simulink model "Demo_DSRC_DNPW_cs"  (Simulink 7.6)
settings: Solver=ode5  SolverMode=SingleTasking  StartTime=0.0  StopTime=5  FixedStep=1/20  RelTol=1e-3
model workspace (MAT data in the model file):
  mbox_table : struct (value not decoded)
  model_closed = 0
  sim_status = 0
PreLoadFcn:
  | check_NUTS_defined;
  | 
  | assignin('base',['model_closed_' bdroot],false);
InitFcn:
  | PreScanExperimentInitFcn(bdroot)
StopFcn:
  | PreScanExperimentStopFcn(bdroot)
undefined symbols (not defined in the file): DiscIntNeverNeededParam, spare_1, spare_10, spare_11, spare_12, spare_13, spare_14, spare_15, spare_16, spare_17, spare_18, spare_19, spare_2, spare_3, spare_4, spare_5, spare_6, spare_7, spare_8, spare_9
libraries: PreScanSimulinkLibrary x29, PreScanUsefulBlocks x11, simulink x9, simulink_extras x2
(part 1 of 6)
CloseFcn:
  | evalin('base',['clear model_closed_' bdroot]);
settings Model: Creator=PRESCAN  LastModifiedBy=buildbot
settings OptimizationCC: InitFltsAndDblsToZero=on
settings DebuggingCC: SaveWithParameterizedLinksMsg=none  SignalResolutionControl=TryResolveAllWithWarning  SolverPrmCheckMsg=none  MultiTaskDSMMsg=warning  MultiTaskCondExecSysMsg=none
settings SFSimCC: SimParseCustomCode=off
settings RTWCC: IncludeERTFirstTime=on
settings GRTTargetCC: TargetFcnLib=ansi_tfl_tmw.mat

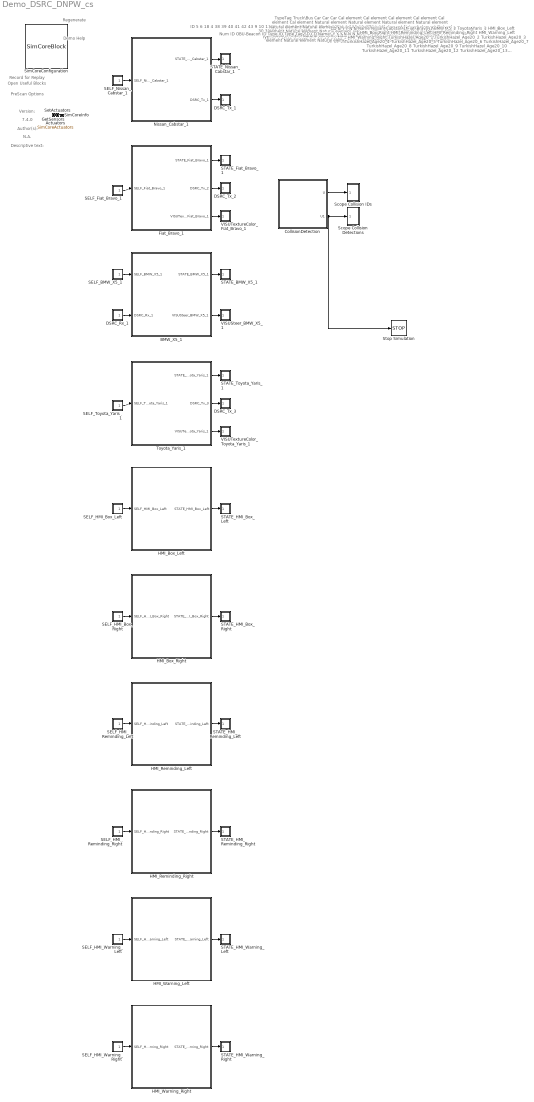
== system Demo_DSRC_DNPW_cs ==
  note: Demo Help
  note: Regenerate
  note: Record for Replay
  note: Open Useful Blocks
  note: PreScan Options
  note: Version:
  note: 7.4.0
  note: Author(s):
  note: N.A.
  note: Descriptive text:
  note: ID
      |
      | 5
      | 6
      | 18
      | 4
      | 38
      | 39
      | 40
      | 41
      | 42
      | 43
      | 9
      | 10
      | 11
      | 12
      | 13
      | 14
      | 15
      | 16
      | 17
      | 19
      | 20
      | 21
      | 22
      | 23
      | 24
      | 25
      | 26
      | 27
      | 28
      | 29
      | 30
      | 31
      | 32
      | 33
      | 34
      | 35
      | 36
      | 37
  note: OBU-Beacon ID
  note: TypeID
      |
      | 3
      | 1
      | 1
      | 1
      | 5
      | 5
      | 5
      | 5
      | 5
      | 5
      | 13
      | 13
      | 13
      | 13
      | 13
      | 13
      | 13
      | 13
      | 13
      | 13
      | 13
      | 13
      | 13
      | 13
      | 13
      | 13
      | 13
      | 13
      | 13
      | 13
      | 13
      | 13
      | 13
      | 13
      | 13
      | 13
      | 13
      | 13
  note: TypeTag
      |
      | Truck\Bus
      | Car
      | Car
      | Car
      | Cal element
      | Cal element
      | Cal element
      | Cal element
      | Cal element
      | Cal element
      | Natural element
      | Natural element
      | Natural element
      | Natural element
      | Natural element
      | Natural element
      | Natural element
      | Natural element
      | Natural element
      | Natural element
      | Natural element
      | Natural element
      | Natural element
      | Natural element
      | Natural element
      | Natural element
      | Natural element
      | Natural element
      | Natural element
      | Natural element
      | Natural element
      | Natural element
      | Natural element
      | Natural element
      | Natural element
      | Natural element
      | Natural element
      | Natural element
  note: SD
      |
      | Y
      | Y
      | Y
      | Y
      | N
      | N
      | N
      | N
      | N
      | N
      | Y
      | Y
      | Y
      | Y
      | Y
      | Y
      | Y
      | Y
      | Y
      | Y
      | Y
      | Y
      | Y
      | Y
      | Y
      | Y
      | Y
      | Y
      | Y
      | Y
      | Y
      | Y
      | Y
      | Y
      | Y
      | Y
      | Y
      | Y
  note: CD
      |
      | N
      | Y
      | Y
      | N
      | N
      | N
      | N
      | N
      | N
      | N
      | N
      | N
      | N
      | N
      | N
      | N
      | N
      | N
      | N
      | N
      | N
      | N
      | N
      | N
      | N
      | N
      | N
      | N
      | N
      | N
      | N
      | N
      | N
      | N
      | N
      | N
      | N
      | N
  note: Name
      |
      | Nissan_Cabstar_1
      | Fiat_Bravo_1
      | BMW_X5_1
      | Toyota_Yaris_1
      | HMI_Box_Left
      | HMI_Box_Right
      | HMI_Reminding_Left
      | HMI_Reminding_Right
      | HMI_Warning_Left
      | HMI_Warning_Right
      | TurkishHazel_Age20_1
      | TurkishHazel_Age20_2
      | TurkishHazel_Age20_3
      | TurkishHazel_Age20_4
      | TurkishHazel_Age20_5
      | TurkishHazel_Age20_6
      | TurkishHazel_Age20_7
      | TurkishHazel_Age20_8
      | TurkishHazel_Age20_9
      | TurkishHazel_Age20_10
      | TurkishHazel_Age20_11
      | TurkishHazel_Age20_12
      | TurkishHazel_Age20_13
      | TurkishHazel_Age20_14
      | TurkishHazel_Age20_15
      | TurkishHazel_Age20_16
      | TurkishHazel_Age20_17
      | TurkishHazel_Age20_18
      | TurkishHazel_Age20_19
      | TurkishHazel_Age20_20
      | TurkishHazel_Age20_21
      | TurkishHazel_Age20_22
      | TurkishHazel_Age20_23
      | TurkishHazel_Age20_24
      | TurkishHazel_Age20_25
      | TurkishHazel_Age20_26
      | TurkishHazel_Age20_27
      | TurkishHazel_Age20_28
  note: Num ID OBU-Beacon ID Type ID Type Tag SD CD Name
  Actuators : DataStoreMemory  Tag=Actuators  DataStoreName=SimCoreActuators  InitialValue=zeros(236,1)
      settings: DeleteFcn=PreScanBlockDeleteFcn;
  BMW_X5_1 : Subsystem  Tag=WorldObjectSubSystem  InitFcn=UniqueId = '51';
      mask Display: image(imread('BMW_X5.jpg'));color('white');text(0,0,' ID=18\n')
  CollisionDetection : Subsystem  Tag=CollisionDetection  Priority=3  mask(PreScan Source Block: CollisionDetection){PortName=CollisionDetection, PortIndex=0, PortWidth=10, TimeStep=1/20}
      mask prompts: PortName "Auto-Assigned: Port Name [-]"; PortIndex "Auto-Assigned: Port Index [-]"; PortWidth "Auto-Assigned: Port Dimensions"; TimeStep "Auto-Assigned: Upload Period [s]"
      mask help:
      | The SELF port shows (state) information of the actor itself. The outputs are position in the experiment's axis system and the GPS coordinates, and the object's absolute velocity and compass heading.
      |
      | For more information, please click Help.
      settings: DeleteFcn=PreScanBlockDeleteFcn;
      mask Help: eval('openHelp(811)')
      mask Display: image(imread('crash.jpg'))
  DSRC_Rx_1 : Subsystem  Tag=DSRC_R  Priority=3  mask(PreScan Source Block: DSRC Receiver){NrEntitiesOut=3, PortName=DSRC_Rx_1, PortIndex=34, PortWidth=141, TimeStep=1/20}
      mask prompts: NrEntitiesOut "User Specified: # of Visible Actors"; PortName "Auto Assigned: Port Name [-]"; PortIndex "Auto Assigned: Index [-]"; PortWidth "Auto Assigned: Port Dimensions [-]"; TimeStep "Auto Assigned: Upload Period [s]"
      mask help:
      | Using the DSRC Receiver (R) and Transmitter (T) information between actors can be exchanged.
      |
      | The DSRC Reciever receives actor information.
      |
      | For more information, please click Help.
      settings: DeleteFcn=PreScanBlockDeleteFcn;
      mask Help: eval('openHelp(473)')
      mask Display: image(imread('DSRCReceiver.png'))
  DSRC_Tx_1 : Subsystem  Tag=DSRC_T  Priority=0  mask(PreScan Sink Block: DSRC_T){PortName=DSRC_Tx_1, PortIndex=15, PortWidth=24, TimeStep=1/20}
      mask prompts: PortName "Auto Assigned: Port Name [-]"; PortIndex "Auto Assigned: Index [-]"; PortWidth "Auto Assigned: Port Dimensions [-]"; TimeStep "Auto Assigned: Upload Period [s]"
      mask help:
      | Using the DSRC Receiver and Transmitter information between actors can be exchanged.
      |
      | The DSRC Transmitter receives actors information.
      |
      | For more information, please click Help.
      settings: DeleteFcn=PreScanBlockDeleteFcn;
      mask Help: eval('openHelp(473)')
      mask Display: image(imread('DSRCTransmitter.png'))
  DSRC_Tx_2 : Subsystem  Tag=DSRC_T  Priority=0  mask(PreScan Sink Block: DSRC_T){PortName=DSRC_Tx_2, PortIndex=54, PortWidth=24, TimeStep=1/20}
      mask prompts: PortName "Auto Assigned: Port Name [-]"; PortIndex "Auto Assigned: Index [-]"; PortWidth "Auto Assigned: Port Dimensions [-]"; TimeStep "Auto Assigned: Upload Period [s]"
      mask help:
      | Using the DSRC Receiver and Transmitter information between actors can be exchanged.
      |
      | The DSRC Transmitter receives actors information.
      |
      | For more information, please click Help.
      settings: DeleteFcn=PreScanBlockDeleteFcn;
      mask Help: eval('openHelp(473)')
      mask Display: image(imread('DSRCTransmitter.png'))
  DSRC_Tx_3 : Subsystem  Tag=DSRC_T  Priority=0  mask(PreScan Sink Block: DSRC_T){PortName=DSRC_Tx_3, PortIndex=119, PortWidth=24, TimeStep=1/20}
      mask prompts: PortName "Auto Assigned: Port Name [-]"; PortIndex "Auto Assigned: Index [-]"; PortWidth "Auto Assigned: Port Dimensions [-]"; TimeStep "Auto Assigned: Upload Period [s]"
      mask help:
      | Using the DSRC Receiver and Transmitter information between actors can be exchanged.
      |
      | The DSRC Transmitter receives actors information.
      |
      | For more information, please click Help.
      settings: DeleteFcn=PreScanBlockDeleteFcn;
      mask Help: eval('openHelp(473)')
      mask Display: image(imread('DSRCTransmitter.png'))
  Fiat_Bravo_1 : Subsystem  Tag=WorldObjectSubSystem  InitFcn=UniqueId = '21';
      mask Display: image(imread('Fiat_Bravo.jpg'));color('white');text(0,0,' ID=6\n')
  GetSensors : Subsystem  Tag=GetSensors  Priority=2  mask(PreScan Simulation Core Block){NrOfSensors=231, TimeStep=1/20}
      mask prompts: NrOfSensors "Number of sensor values"; TimeStep "Timestep [s]"
      mask help:
      | Please do not remove this block from the PreScan compilation sheet,
      | as it contains essential configuration parameters for a PreScan simulation.
      settings: DeleteFcn=PreScanBlockDeleteFcn;
  HMI_Box_Left : Subsystem  Tag=WorldObjectSubSystem  InitFcn=UniqueId = '84';
      mask Display: image(imread('Box.jpg'));color('white');text(0,0,' ID=38\n')
  HMI_Box_Right : Subsystem  Tag=WorldObjectSubSystem  InitFcn=UniqueId = '85';
      mask Display: image(imread('Box.jpg'));color('white');text(0,0,' ID=39\n')
  HMI_Reminding_Left : Subsystem  Tag=WorldObjectSubSystem  InitFcn=UniqueId = '86';
      mask Display: image(imread('Sphere.jpg'));color('white');text(0,0,' ID=40\n')
  HMI_Reminding_Right : Subsystem  Tag=WorldObjectSubSystem  InitFcn=UniqueId = '87';
      mask Display: image(imread('Sphere.jpg'));color('white');text(0,0,' ID=41\n')
  HMI_Warning_Left : Subsystem  Tag=WorldObjectSubSystem  InitFcn=UniqueId = '88';
      mask Display: image(imread('Sphere.jpg'));color('white');text(0,0,' ID=42\n')
  HMI_Warning_Right : Subsystem  Tag=WorldObjectSubSystem  InitFcn=UniqueId = '89';
      mask Display: image(imread('Sphere.jpg'));color('white');text(0,0,' ID=43\n')
  Nissan_Cabstar_1 : Subsystem  Tag=WorldObjectSubSystem  InitFcn=UniqueId = '19';
      mask Display: image(imread('Nissan_Cabstar.jpg'));color('white');text(0,0,' ID=5\n')
  SELF_BMW_X5_1 : Subsystem  Tag=SELF  Priority=3  mask(PreScan Source Block: SELF){PortName=SELF_BMW_X5_1, PortIndex=26, PortWidth=8, TimeStep=1/20}
      mask prompts: PortName "Auto-Assigned: Port Name [-]"; PortIndex "Auto-Assigned: Port Index [-]"; PortWidth "Auto-Assigned: Port Dimensions"; TimeStep "Auto-Assigned: Upload Period [s]"
      mask help:
      | The SELF port shows (state) information of the actor itself. The outputs are position in the experiment's axis system and the GPS coordinates, and the object's absolute velocity and compass heading.
      |
      | For more information, please click Help.
      settings: DeleteFcn=PreScanBlockDeleteFcn;
      mask Help: eval('openHelp(462)')
      mask Display: image(imread('GPS.png'))
  SELF_Fiat_Bravo_1 : Subsystem  Tag=SELF  Priority=3  mask(PreScan Source Block: SELF){PortName=SELF_Fiat_Bravo_1, PortIndex=18, PortWidth=8, TimeStep=1/20}
      mask prompts: PortName "Auto-Assigned: Port Name [-]"; PortIndex "Auto-Assigned: Port Index [-]"; PortWidth "Auto-Assigned: Port Dimensions"; TimeStep "Auto-Assigned: Upload Period [s]"
      mask help:
      | The SELF port shows (state) information of the actor itself. The outputs are position in the experiment's axis system and the GPS coordinates, and the object's absolute velocity and compass heading.
      |
      | For more information, please click Help.
      settings: DeleteFcn=PreScanBlockDeleteFcn;
      mask Help: eval('openHelp(462)')
      mask Display: image(imread('GPS.png'))
  SELF_HMI_Box_Left : Subsystem  Tag=SELF  Priority=3  mask(PreScan Source Block: SELF){PortName=SELF_HMI_Box_Left, PortIndex=183, PortWidth=8, TimeStep=1/20}
      mask prompts: PortName "Auto-Assigned: Port Name [-]"; PortIndex "Auto-Assigned: Port Index [-]"; PortWidth "Auto-Assigned: Port Dimensions"; TimeStep "Auto-Assigned: Upload Period [s]"
      mask help:
      | The SELF port shows (state) information of the actor itself. The outputs are position in the experiment's axis system and the GPS coordinates, and the object's absolute velocity and compass heading.
      |
      | For more information, please click Help.
      settings: DeleteFcn=PreScanBlockDeleteFcn;
      mask Help: eval('openHelp(462)')
      mask Display: image(imread('GPS.png'))
  SELF_HMI_Box_Right : Subsystem  Tag=SELF  Priority=3  mask(PreScan Source Block: SELF){PortName=SELF_HMI_Box_Right, PortIndex=191, PortWidth=8, TimeStep=1/20}
      mask prompts: PortName "Auto-Assigned: Port Name [-]"; PortIndex "Auto-Assigned: Port Index [-]"; PortWidth "Auto-Assigned: Port Dimensions"; TimeStep "Auto-Assigned: Upload Period [s]"
      mask help:
      | The SELF port shows (state) information of the actor itself. The outputs are position in the experiment's axis system and the GPS coordinates, and the object's absolute velocity and compass heading.
      |
      | For more information, please click Help.
      settings: DeleteFcn=PreScanBlockDeleteFcn;
      mask Help: eval('openHelp(462)')
      mask Display: image(imread('GPS.png'))
  SELF_HMI_Reminding_Left : Subsystem  Tag=SELF  Priority=3  mask(PreScan Source Block: SELF){PortName=SELF_HMI_Reminding_Left, PortIndex=199, PortWidth=8, TimeStep=1/20}
      mask prompts: PortName "Auto-Assigned: Port Name [-]"; PortIndex "Auto-Assigned: Port Index [-]"; PortWidth "Auto-Assigned: Port Dimensions"; TimeStep "Auto-Assigned: Upload Period [s]"
      mask help:
      | The SELF port shows (state) information of the actor itself. The outputs are position in the experiment's axis system and the GPS coordinates, and the object's absolute velocity and compass heading.
      |
      | For more information, please click Help.
      settings: DeleteFcn=PreScanBlockDeleteFcn;
      mask Help: eval('openHelp(462)')
      mask Display: image(imread('GPS.png'))
  SELF_HMI_Reminding_Right : Subsystem  Tag=SELF  Priority=3  mask(PreScan Source Block: SELF){PortName=SELF_HMI_Reminding_Right, PortIndex=207, PortWidth=8, TimeStep=1/20}
      mask prompts: PortName "Auto-Assigned: Port Name [-]"; PortIndex "Auto-Assigned: Port Index [-]"; PortWidth "Auto-Assigned: Port Dimensions"; TimeStep "Auto-Assigned: Upload Period [s]"
      mask help:
      | The SELF port shows (state) information of the actor itself. The outputs are position in the experiment's axis system and the GPS coordinates, and the object's absolute velocity and compass heading.
      |
      | For more information, please click Help.
      settings: DeleteFcn=PreScanBlockDeleteFcn;
      mask Help: eval('openHelp(462)')
      mask Display: image(imread('GPS.png'))
  SELF_HMI_Warning_Left : Subsystem  Tag=SELF  Priority=3  mask(PreScan Source Block: SELF){PortName=SELF_HMI_Warning_Left, PortIndex=215, PortWidth=8, TimeStep=1/20}
      mask prompts: PortName "Auto-Assigned: Port Name [-]"; PortIndex "Auto-Assigned: Port Index [-]"; PortWidth "Auto-Assigned: Port Dimensions"; TimeStep "Auto-Assigned: Upload Period [s]"
      mask help:
      | The SELF port shows (state) information of the actor itself. The outputs are position in the experiment's axis system and the GPS coordinates, and the object's absolute velocity and compass heading.
      |
      | For more information, please click Help.
      settings: DeleteFcn=PreScanBlockDeleteFcn;
      mask Help: eval('openHelp(462)')
      mask Display: image(imread('GPS.png'))
  SELF_HMI_Warning_Right : Subsystem  Tag=SELF  Priority=3  mask(PreScan Source Block: SELF){PortName=SELF_HMI_Warning_Right, PortIndex=223, PortWidth=8, TimeStep=1/20}
      mask prompts: PortName "Auto-Assigned: Port Name [-]"; PortIndex "Auto-Assigned: Port Index [-]"; PortWidth "Auto-Assigned: Port Dimensions"; TimeStep "Auto-Assigned: Upload Period [s]"
      mask help:
      | The SELF port shows (state) information of the actor itself. The outputs are position in the experiment's axis system and the GPS coordinates, and the object's absolute velocity and compass heading.
      |
      | For more information, please click Help.
      settings: DeleteFcn=PreScanBlockDeleteFcn;
      mask Help: eval('openHelp(462)')
      mask Display: image(imread('GPS.png'))
  SELF_Nissan_Cabstar_1 : Subsystem  Tag=SELF  Priority=3  mask(PreScan Source Block: SELF){PortName=SELF_Nissan_Cabstar_1, PortIndex=10, PortWidth=8, TimeStep=1/20}
      mask prompts: PortName "Auto-Assigned: Port Name [-]"; PortIndex "Auto-Assigned: Port Index [-]"; PortWidth "Auto-Assigned: Port Dimensions"; TimeStep "Auto-Assigned: Upload Period [s]"
      mask help:
      | The SELF port shows (state) information of the actor itself. The outputs are position in the experiment's axis system and the GPS coordinates, and the object's absolute velocity and compass heading.
      |
      | For more information, please click Help.
      settings: DeleteFcn=PreScanBlockDeleteFcn;
      mask Help: eval('openHelp(462)')
      mask Display: image(imread('GPS.png'))
  SELF_Toyota_Yaris_1 : Subsystem  Tag=SELF  Priority=3  mask(PreScan Source Block: SELF){PortName=SELF_Toyota_Yaris_1, PortIndex=175, PortWidth=8, TimeStep=1/20}
      mask prompts: PortName "Auto-Assigned: Port Name [-]"; PortIndex "Auto-Assigned: Port Index [-]"; PortWidth "Auto-Assigned: Port Dimensions"; TimeStep "Auto-Assigned: Upload Period [s]"
      mask help:
      | The SELF port shows (state) information of the actor itself. The outputs are position in the experiment's axis system and the GPS coordinates, and the object's absolute velocity and compass heading.
      |
      | For more information, please click Help.
      settings: DeleteFcn=PreScanBlockDeleteFcn;
      mask Help: eval('openHelp(462)')
      mask Display: image(imread('GPS.png'))
  STATE_BMW_X5_1 : Subsystem  Tag=State  Priority=0  mask(PreScan Sink Block: State){x0=24.209174789062494, y0=46.159446700000011, z0=0.69, Roll0=0, Pitch0=0, Yaw0=7.0164775638926606E-15, TimeStep=1/20}
      mask prompts: x0 "Ini x-position VEHICLE wrt GLOBAL axis system [m]"; y0 "Ini y-position VEHICLE wrt GLOBAL axis system [m]"; z0 "Ini z-position VEHICLE wrt GLOBAL axis system [m]"; Roll0 "Ini roll-angle BODY wrt VEHICLE axis system [deg]"; Pitch0 "Ini pitch-angle BODY wrt VEHICLE axis system [deg]"; Yaw0 "Ini yaw-angle VEHICLE wrt GLOBAL axis system [deg]"; TimeStep "Time Step [s]"
      mask help:
      | The Actor State contains a vector signal of size (9x1), containing the following signals:
      |
      | -  Position                  (x,y,z)                                     [m]
      | -  Velocity                  (vx,vy,vz)                               [m/s]
      | -  Angles                    (Roll, Pitch, Yaw)                   [rad]
      |
      | The Actor state is defined in the global axis system.
      | The state is superponed on the Initial position defined in the GUI.
      |
      | For more information, please click Help.
      settings: DeleteFcn=PreScanBlockDeleteFcn;
      mask Help: eval('openHelp(222)')
      mask Display: image(imread('State.png'))
  STATE_Fiat_Bravo_1 : Subsystem  Tag=State  Priority=0  mask(PreScan Sink Block: State){x0=242.54259629004468, y0=49.399995071782, z0=0.58, Roll0=0, Pitch0=0, Yaw0=180.0000065161471, TimeStep=1/20}
      mask prompts: x0 "Ini x-position VEHICLE wrt GLOBAL axis system [m]"; y0 "Ini y-position VEHICLE wrt GLOBAL axis system [m]"; z0 "Ini z-position VEHICLE wrt GLOBAL axis system [m]"; Roll0 "Ini roll-angle BODY wrt VEHICLE axis system [deg]"; Pitch0 "Ini pitch-angle BODY wrt VEHICLE axis system [deg]"; Yaw0 "Ini yaw-angle VEHICLE wrt GLOBAL axis system [deg]"; TimeStep "Time Step [s]"
      mask help:
      | The Actor State contains a vector signal of size (9x1), containing the following signals:
      |
      | -  Position                  (x,y,z)                                     [m]
      | -  Velocity                  (vx,vy,vz)                               [m/s]
      | -  Angles                    (Roll, Pitch, Yaw)                   [rad]
      |
      | The Actor state is defined in the global axis system.
      | The state is superponed on the Initial position defined in the GUI.
      |
      | For more information, please click Help.
      settings: DeleteFcn=PreScanBlockDeleteFcn;
      mask Help: eval('openHelp(222)')
      mask Display: image(imread('State.png'))
  STATE_HMI_Box_Left : Subsystem  Tag=State  Priority=0  mask(PreScan Sink Block: State){x0=24.2091747890625, y0=46.1594467, z0=0.69, Roll0=0, Pitch0=0, Yaw0=0, TimeStep=1/20}
      mask prompts: x0 "Ini x-position VEHICLE wrt GLOBAL axis system [m]"; y0 "Ini y-position VEHICLE wrt GLOBAL axis system [m]"; z0 "Ini z-position VEHICLE wrt GLOBAL axis system [m]"; Roll0 "Ini roll-angle BODY wrt VEHICLE axis system [deg]"; Pitch0 "Ini pitch-angle BODY wrt VEHICLE axis system [deg]"; Yaw0 "Ini yaw-angle VEHICLE wrt GLOBAL axis system [deg]"; TimeStep "Time Step [s]"
      mask help:
      | The Actor State contains a vector signal of size (9x1), containing the following signals:
      |
      | -  Position                  (x,y,z)                                     [m]
      | -  Velocity                  (vx,vy,vz)                               [m/s]
      | -  Angles                    (Roll, Pitch, Yaw)                   [rad]
      |
      | The Actor state is defined in the global axis system.
      | The state is superponed on the Initial position defined in the GUI.
      |
      | For more information, please click Help.
      settings: DeleteFcn=PreScanBlockDeleteFcn;
      mask Help: eval('openHelp(222)')
      mask Display: image(imread('State.png'))
  STATE_HMI_Box_Right : Subsystem  Tag=State  Priority=0  mask(PreScan Sink Block: State){x0=24.2091747890625, y0=46.1594467, z0=0.69, Roll0=0, Pitch0=0, Yaw0=0, TimeStep=1/20}
      mask prompts: x0 "Ini x-position VEHICLE wrt GLOBAL axis system [m]"; y0 "Ini y-position VEHICLE wrt GLOBAL axis system [m]"; z0 "Ini z-position VEHICLE wrt GLOBAL axis system [m]"; Roll0 "Ini roll-angle BODY wrt VEHICLE axis system [deg]"; Pitch0 "Ini pitch-angle BODY wrt VEHICLE axis system [deg]"; Yaw0 "Ini yaw-angle VEHICLE wrt GLOBAL axis system [deg]"; TimeStep "Time Step [s]"
      mask help:
      | The Actor State contains a vector signal of size (9x1), containing the following signals:
      |
      | -  Position                  (x,y,z)                                     [m]
      | -  Velocity                  (vx,vy,vz)                               [m/s]
      | -  Angles                    (Roll, Pitch, Yaw)                   [rad]
      |
      | The Actor state is defined in the global axis system.
      | The state is superponed on the Initial position defined in the GUI.
      |
      | For more information, please click Help.
      settings: DeleteFcn=PreScanBlockDeleteFcn;
      mask Help: eval('openHelp(222)')
      mask Display: image(imread('State.png'))
  STATE_HMI_Reminding_Left : Subsystem  Tag=State  Priority=0  mask(PreScan Sink Block: State){x0=24.2091747890625, y0=46.1594467, z0=0.69, Roll0=0, Pitch0=0, Yaw0=0, TimeStep=1/20}
      mask prompts: x0 "Ini x-position VEHICLE wrt GLOBAL axis system [m]"; y0 "Ini y-position VEHICLE wrt GLOBAL axis system [m]"; z0 "Ini z-position VEHICLE wrt GLOBAL axis system [m]"; Roll0 "Ini roll-angle BODY wrt VEHICLE axis system [deg]"; Pitch0 "Ini pitch-angle BODY wrt VEHICLE axis system [deg]"; Yaw0 "Ini yaw-angle VEHICLE wrt GLOBAL axis system [deg]"; TimeStep "Time Step [s]"
      mask help:
      | The Actor State contains a vector signal of size (9x1), containing the following signals:
      |
      | -  Position                  (x,y,z)                                     [m]
      | -  Velocity                  (vx,vy,vz)                               [m/s]
      | -  Angles                    (Roll, Pitch, Yaw)                   [rad]
      |
      | The Actor state is defined in the global axis system.
      | The state is superponed on the Initial position defined in the GUI.
      |
      | For more information, please click Help.
      settings: DeleteFcn=PreScanBlockDeleteFcn;
      mask Help: eval('openHelp(222)')
      mask Display: image(imread('State.png'))
  STATE_HMI_Reminding_Right : Subsystem  Tag=State  Priority=0  mask(PreScan Sink Block: State){x0=24.2091747890625, y0=46.1594467, z0=0.69, Roll0=0, Pitch0=0, Yaw0=0, TimeStep=1/20}
      mask prompts: x0 "Ini x-position VEHICLE wrt GLOBAL axis system [m]"; y0 "Ini y-position VEHICLE wrt GLOBAL axis system [m]"; z0 "Ini z-position VEHICLE wrt GLOBAL axis system [m]"; Roll0 "Ini roll-angle BODY wrt VEHICLE axis system [deg]"; Pitch0 "Ini pitch-angle BODY wrt VEHICLE axis system [deg]"; Yaw0 "Ini yaw-angle VEHICLE wrt GLOBAL axis system [deg]"; TimeStep "Time Step [s]"
      mask help:
      | The Actor State contains a vector signal of size (9x1), containing the following signals:
      |
      | -  Position                  (x,y,z)                                     [m]
      | -  Velocity                  (vx,vy,vz)                               [m/s]
      | -  Angles                    (Roll, Pitch, Yaw)                   [rad]
      |
      | The Actor state is defined in the global axis system.
      | The state is superponed on the Initial position defined in the GUI.
      |
      | For more information, please click Help.
      settings: DeleteFcn=PreScanBlockDeleteFcn;
      mask Help: eval('openHelp(222)')
      mask Display: image(imread('State.png'))
  STATE_HMI_Warning_Left : Subsystem  Tag=State  Priority=0  mask(PreScan Sink Block: State){x0=24.2091747890625, y0=46.1594467, z0=0.69, Roll0=0, Pitch0=0, Yaw0=0, TimeStep=1/20}
      mask prompts: x0 "Ini x-position VEHICLE wrt GLOBAL axis system [m]"; y0 "Ini y-position VEHICLE wrt GLOBAL axis system [m]"; z0 "Ini z-position VEHICLE wrt GLOBAL axis system [m]"; Roll0 "Ini roll-angle BODY wrt VEHICLE axis system [deg]"; Pitch0 "Ini pitch-angle BODY wrt VEHICLE axis system [deg]"; Yaw0 "Ini yaw-angle VEHICLE wrt GLOBAL axis system [deg]"; TimeStep "Time Step [s]"
      mask help:
      | The Actor State contains a vector signal of size (9x1), containing the following signals:
      |
      | -  Position                  (x,y,z)                                     [m]
      | -  Velocity                  (vx,vy,vz)                               [m/s]
      | -  Angles                    (Roll, Pitch, Yaw)                   [rad]
      |
      | The Actor state is defined in the global axis system.
      | The state is superponed on the Initial position defined in the GUI.
      |
      | For more information, please click Help.
      settings: DeleteFcn=PreScanBlockDeleteFcn;
      mask Help: eval('openHelp(222)')
      mask Display: image(imread('State.png'))
  STATE_HMI_Warning_Right : Subsystem  Tag=State  Priority=0  mask(PreScan Sink Block: State){x0=24.2091747890625, y0=46.1594467, z0=0.69, Roll0=0, Pitch0=0, Yaw0=0, TimeStep=1/20}
      mask prompts: x0 "Ini x-position VEHICLE wrt GLOBAL axis system [m]"; y0 "Ini y-position VEHICLE wrt GLOBAL axis system [m]"; z0 "Ini z-position VEHICLE wrt GLOBAL axis system [m]"; Roll0 "Ini roll-angle BODY wrt VEHICLE axis system [deg]"; Pitch0 "Ini pitch-angle BODY wrt VEHICLE axis system [deg]"; Yaw0 "Ini yaw-angle VEHICLE wrt GLOBAL axis system [deg]"; TimeStep "Time Step [s]"
      mask help:
      | The Actor State contains a vector signal of size (9x1), containing the following signals:
      |
      | -  Position                  (x,y,z)                                     [m]
      | -  Velocity                  (vx,vy,vz)                               [m/s]
      | -  Angles                    (Roll, Pitch, Yaw)                   [rad]
      |
      | The Actor state is defined in the global axis system.
      | The state is superponed on the Initial position defined in the GUI.
      |
      | For more information, please click Help.
      settings: DeleteFcn=PreScanBlockDeleteFcn;
      mask Help: eval('openHelp(222)')
      mask Display: image(imread('State.png'))
  STATE_Nissan_Cabstar_1 : Subsystem  Tag=State  Priority=0  mask(PreScan Sink Block: State){x0=60.875884988087634, y0=46.5, z0=0.88, Roll0=0, Pitch0=0, Yaw0=6.5161470956809362E-06, TimeStep=1/20}
      mask prompts: x0 "Ini x-position VEHICLE wrt GLOBAL axis system [m]"; y0 "Ini y-position VEHICLE wrt GLOBAL axis system [m]"; z0 "Ini z-position VEHICLE wrt GLOBAL axis system [m]"; Roll0 "Ini roll-angle BODY wrt VEHICLE axis system [deg]"; Pitch0 "Ini pitch-angle BODY wrt VEHICLE axis system [deg]"; Yaw0 "Ini yaw-angle VEHICLE wrt GLOBAL axis system [deg]"; TimeStep "Time Step [s]"
      mask help:
      | The Actor State contains a vector signal of size (9x1), containing the following signals:
      |
      | -  Position                  (x,y,z)                                     [m]
      | -  Velocity                  (vx,vy,vz)                               [m/s]
      | -  Angles                    (Roll, Pitch, Yaw)                   [rad]
      |
      | The Actor state is defined in the global axis system.
      | The state is superponed on the Initial position defined in the GUI.
      |
      | For more information, please click Help.
      settings: DeleteFcn=PreScanBlockDeleteFcn;
      mask Help: eval('openHelp(222)')
      mask Display: image(imread('State.png'))
  STATE_Toyota_Yaris_1 : Subsystem  Tag=State  Priority=0  mask(PreScan Sink Block: State){x0=111.62059801670154, y0=43.500005743275182, z0=0.57, Roll0=0, Pitch0=0, Yaw0=6.5161471026974123E-06, TimeStep=1/20}
      mask prompts: x0 "Ini x-position VEHICLE wrt GLOBAL axis system [m]"; y0 "Ini y-position VEHICLE wrt GLOBAL axis system [m]"; z0 "Ini z-position VEHICLE wrt GLOBAL axis system [m]"; Roll0 "Ini roll-angle BODY wrt VEHICLE axis system [deg]"; Pitch0 "Ini pitch-angle BODY wrt VEHICLE axis system [deg]"; Yaw0 "Ini yaw-angle VEHICLE wrt GLOBAL axis system [deg]"; TimeStep "Time Step [s]"
      mask help:
      | The Actor State contains a vector signal of size (9x1), containing the following signals:
      |
      | -  Position                  (x,y,z)                                     [m]
      | -  Velocity                  (vx,vy,vz)                               [m/s]
      | -  Angles                    (Roll, Pitch, Yaw)                   [rad]
      |
      | The Actor state is defined in the global axis system.
      | The state is superponed on the Initial position defined in the GUI.
      |
      | For more information, please click Help.
      settings: DeleteFcn=PreScanBlockDeleteFcn;
      mask Help: eval('openHelp(222)')
      mask Display: image(imread('State.png'))
  Scope Collision Detections : Subsystem  Tag=Scope Collision Detections
      settings: DeleteFcn=PreScanBlockDeleteFcn;
      settings: OpenFcn=|
      | blockname=[get_param(gcb,'Parent'),'/',get_param(gcb,'Name')];
      | subblockname=[blockname,'/Collision Detections'];
      | open_system(subblockname);
      | close_system(blockname);
      mask Display:
      | plot([0.5 9.5 9.5 0.5 0.5],[5 5 9 9 5])
      | plot(0,0)
      | plot(10,10)
      | text(0,1,'P+')
  Scope Collision IDs : Subsystem  Tag=Scope Collision IDs
      settings: DeleteFcn=PreScanBlockDeleteFcn;
      settings: OpenFcn=|
      | blockname=[get_param(gcb,'Parent'),'/',get_param(gcb,'Name')];
      | subblockname=[blockname,'/Collision IDs'];
      | open_system(subblockname);
      | close_system(blockname);
      mask Display:
      | plot([0.5 9.5 9.5 0.5 0.5],[5 5 9 9 5])
      | plot(0,0)
      | plot(10,10)
      | text(0,1,'P+')
  SetActuators : Subsystem  Tag=SetActuators  Priority=1  mask(PreScan Simulation Core Block){TimeStep=1/20, NrOfActuators=236}
      mask prompts: TimeStep "Timestep [s]"; NrOfActuators "Number of actuator values"
      mask help:
      | Please do not remove this block from the PreScan compilation sheet,
      | as it contains essential configuration parameters for a PreScan simulation.
      settings: DeleteFcn=PreScanBlockDeleteFcn;
  SimCoreConfiguration : M-S-Function  Tag=SimCoreConfiguration  Description=8EDCDAF3ABFF8DA37C0E4289C387709BD73B99DB21475762D6C7E2C9E51573E2  FunctionName=SimCoreBlock  Parameters=ExperimentXML PortsXML SimulationCore HostName CheckStart EnableLog RfR EnableGPUAccel ShowComputationTime  mask(PreScan Simulation Core Configurator){SimulationCore=NUTS, HostName=0, CheckStart=0, prescanversion='7.4.0', EnableLog=off, RfR=0, EnableGPUAccel=off, ShowComputationTime=off}
      mask prompts: SimulationCore "Simulation Core"; HostName "Simulation Host"; CheckStart "Show START Dialog"; prescanversion "PreScan Version"; EnableLog "Create TA Log"; RfR "Record for Replay"; EnableGPUAccel "Enable GPU Acceleration"; ShowComputationTime "Show ComputationTime Scope"
      mask help:
      | Please do not remove this block from the PreScan compilation sheet,
      | as it contains essential configuration parameter for a PreScan simulation.
      mask init:
      | model = bdroot;
      | ExperimentXML = [model(1:end-3) '.pex'];
      | PortsXML = [model '_ports.pcd'];
      settings: DeleteFcn=PreScanBlockDeleteFcn;  ModelCloseFcn=assignin('base',['model_closed_' bdroot],true);
      mask Help: eval('openHelp(812)')
      mask Display: image(imread('prescanlogo.ico'))
  SimCoreInfo : Subsystem  Tag=SimCoreInfo
  Stop Simulation : Stop
  Toyota_Yaris_1 : Subsystem  Tag=WorldObjectSubSystem  InitFcn=UniqueId = '79';
      mask Display: image(imread('Toyota_Yaris.jpg'));color('white');text(0,0,' ID=4\n')
  VISUSteer_BMW_X5_1 : Subsystem  Tag=VisuSteer  Priority=0
      settings: DeleteFcn=PreScanBlockDeleteFcn;
      mask Type: PreScan Sink Block: VisuSteer
      mask Description:
      | The VisuSteer block provides a way to adapt the orientation of the steering column and steering wheel of a vehicle.
      | 
      | For more information, please click Help.
      mask Help: eval('openHelp(223)')
      mask Display: image(imread('steeringwheel.png'))
  VISUTextureColor_Fiat_Bravo_1 : Subsystem  Tag=VisuTextureColor  Priority=0
      settings: DeleteFcn=PreScanBlockDeleteFcn;
      mask Type: PreScan Sink Block: VisuTextureColor
      mask Description:
      | The Texture Color block provides a way to adapt the color of a vehicle.
      | 
      | For more information, please click Help.
      mask Help: eval('openHelp(230)')
      mask Display: image(imread('TextureColor.png'))
  VISUTextureColor_Toyota_Yaris_1 : Subsystem  Tag=VisuTextureColor  Priority=0
      settings: DeleteFcn=PreScanBlockDeleteFcn;
      mask Type: PreScan Sink Block: VisuTextureColor
      mask Description:
      | The Texture Color block provides a way to adapt the color of a vehicle.
      | 
      | For more information, please click Help.
      mask Help: eval('openHelp(230)')
      mask Display: image(imread('TextureColor.png'))
  wires:
  CollisionDetection/1(U) -> Scope Collision IDs/1(In1)
  CollisionDetection/2(U1) -> Scope Collision Detections/1(In1), Stop Simulation/1
  Nissan_Cabstar_1/1(STATE_Nissan_Cabstar_1) -> STATE_Nissan_Cabstar_1/1(State)
  SELF_Nissan_Cabstar_1/1(U) -> Nissan_Cabstar_1/1(SELF_Nissan_Cabstar_1)
  Nissan_Cabstar_1/2(DSRC_Tx_1) -> DSRC_Tx_1/1(Y)
  Fiat_Bravo_1/1(STATE_Fiat_Bravo_1) -> STATE_Fiat_Bravo_1/1(State)
  SELF_Fiat_Bravo_1/1(U) -> Fiat_Bravo_1/1(SELF_Fiat_Bravo_1)
  Fiat_Bravo_1/2(DSRC_Tx_2) -> DSRC_Tx_2/1(Y)
  Fiat_Bravo_1/3(VISUTextureColor_Fiat_Bravo_1) -> VISUTextureColor_Fiat_Bravo_1/1(TextureColor)
  BMW_X5_1/1(STATE_BMW_X5_1) -> STATE_BMW_X5_1/1(State)
  SELF_BMW_X5_1/1(U) -> BMW_X5_1/1(SELF_BMW_X5_1)
  DSRC_Rx_1/1(U) -> BMW_X5_1/2(DSRC_Rx_1)
  BMW_X5_1/2(VISUSteer_BMW_X5_1) -> VISUSteer_BMW_X5_1/1(Steer)
  Toyota_Yaris_1/1(STATE_Toyota_Yaris_1) -> STATE_Toyota_Yaris_1/1(State)
  SELF_Toyota_Yaris_1/1(U) -> Toyota_Yaris_1/1(SELF_Toyota_Yaris_1)
  Toyota_Yaris_1/2(DSRC_Tx_3) -> DSRC_Tx_3/1(Y)
  Toyota_Yaris_1/3(VISUTextureColor_Toyota_Yaris_1) -> VISUTextureColor_Toyota_Yaris_1/1(TextureColor)
  HMI_Box_Left/1(STATE_HMI_Box_Left) -> STATE_HMI_Box_Left/1(State)
  SELF_HMI_Box_Left/1(U) -> HMI_Box_Left/1(SELF_HMI_Box_Left)
  HMI_Box_Right/1(STATE_HMI_Box_Right) -> STATE_HMI_Box_Right/1(State)
  SELF_HMI_Box_Right/1(U) -> HMI_Box_Right/1(SELF_HMI_Box_Right)
  HMI_Reminding_Left/1(STATE_HMI_Reminding_Left) -> STATE_HMI_Reminding_Left/1(State)
  SELF_HMI_Reminding_Left/1(U) -> HMI_Reminding_Left/1(SELF_HMI_Reminding_Left)
  HMI_Reminding_Right/1(STATE_HMI_Reminding_Right) -> STATE_HMI_Reminding_Right/1(State)
  SELF_HMI_Reminding_Right/1(U) -> HMI_Reminding_Right/1(SELF_HMI_Reminding_Right)
  HMI_Warning_Left/1(STATE_HMI_Warning_Left) -> STATE_HMI_Warning_Left/1(State)
  SELF_HMI_Warning_Left/1(U) -> HMI_Warning_Left/1(SELF_HMI_Warning_Left)
  HMI_Warning_Right/1(STATE_HMI_Warning_Right) -> STATE_HMI_Warning_Right/1(State)
  SELF_HMI_Warning_Right/1(U) -> HMI_Warning_Right/1(SELF_HMI_Warning_Right)
  SetActuators/1(dummy) -> GetSensors/1(dummy)

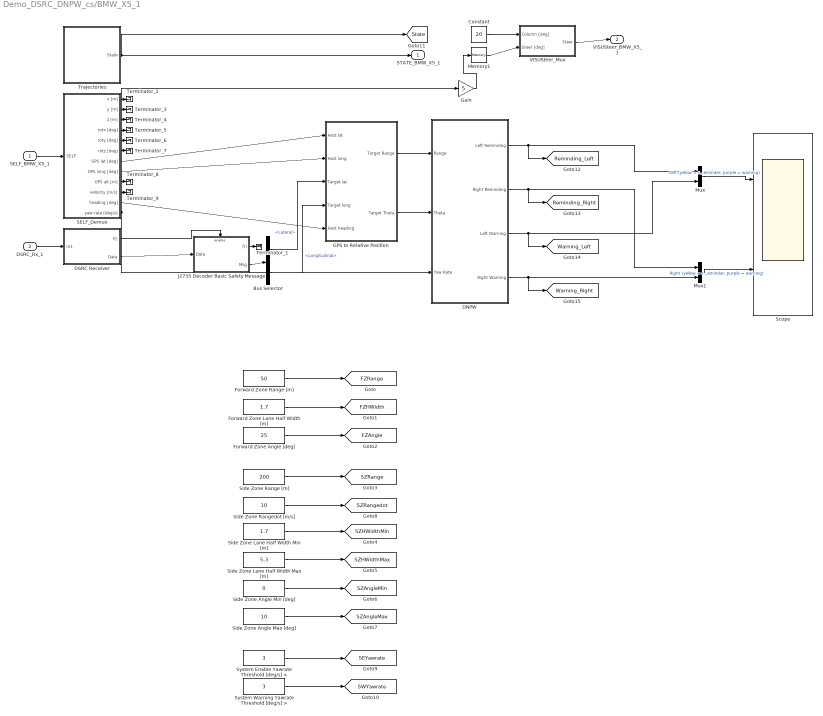
== system Demo_DSRC_DNPW_cs/BMW_X5_1 ==
  SELF_BMW_X5_1 : Inport  Tag=SELFInport
  DSRC_Rx_1 : Inport  Tag=DSRC_RInport  Port=2
  Bus Selector : BusSelector  OutputSignals=Lateral,Longitudinal
  Constant : Constant  Value=20
  DNPW : Subsystem
  DSRC Receiver : Subsystem  Tag=DSRC_Receiver
  Forward Zone Angle [deg] : Constant  Value=25
  Forward Zone Lane Half Width [m] : Constant  Value=1.7
  Forward Zone Range [m] : Constant  Value=50
  GPS to Relative Position : Subsystem
  Gain : Gain  Gain=5
  J2735 Decoder Basic Safety Message : Subsystem  Tag=J2735_Decoder_Basic_Safety_Message
  Memory1 : Memory
  Mux : Mux  Inputs=2
  Mux1 : Mux  Inputs=2
  SELF_Demux : Subsystem  Tag=DemuxSELF
      settings: DeleteFcn=PreScanBlockDeleteFcn;
      mask Type: PreScan Demux Block:
      mask Display:
      | port_label('output',1,'x [m]')
      | port_label('output',2,'y [m]')
      | port_label('output',3,'z [m]','texmode','on')
      | port_label('output',4,'Rotx [deg]','texmode','on')
      | port_label('output',5,'Roty [deg]','texmode','on')
      | port_label('output',6,'Rotz [deg]','texmode','on')
      | port_label('output',7,'GPS lat [deg]','texmode','on')
      | port_label('output',8,'GPS long [deg]','texmode','on')
      | port_label('output',9,'GPS alt [m]','texmode','on')
      | port_label('output',10,'Velocity [m/s]')
      | port_label('output',11,'Heading [deg]')
      | port_label('output',12,'Yaw rate [deg/s]')
  SIde Zone Angle Max [deg] : Constant  Value=10
  SIde Zone Angle Min [deg] : Constant  Value=0
  Scope : Scope  NumInputPorts=2
      settings: YMin=0~0  YMax=2~2
  Side Zone Lane Half Width Max [m] : Constant  Value=5.3
  Side Zone Lane Half Width Min [m] : Constant  Value=1.7
  Side Zone Range [m] : Constant  Value=200
  Side Zone Rangedot [m/s] : Constant  Value=10
  System Enable Yawrate Threshold [deg/s] < : Constant  Value=3
  System Warning Yawrate Threshold [deg/s] > : Constant  Value=3
  Terminator_{1..9} (9 alike) : Terminator
  Trajectories : Subsystem  Tag=Trajectories
      settings: DeleteFcn=PreScanBlockDeleteFcn;
      mask Type: PreScan Source Block: Trajectories
      mask Description:
      | The Trajectory block contains the trajectories defined in the PreScan Experiment Editor. The output of the trajectory block is the (vehicle) State.
      | 
      | For more information, please click Help.
      mask Help: eval('openHelp(312)')
      mask Display: image(imread('Trajectory.png'));
  VISUSteer_Mux : Subsystem  Tag=MuxSteer
      settings: DeleteFcn=PreScanBlockDeleteFcn;
      mask Type: PreScan Mux Block:
  STATE_BMW_X5_1 : Outport  Tag=StateOutport
  VISUSteer_BMW_X5_1 : Outport  Tag=VisuSteerOutport  Port=2  SampleTime=1/20
  tag scope: FZAngle=global, FZHWidth=global, FZRange=global, Reminding_Left=global, Reminding_Right=global, SEYawrate=global, SWYawrate=global, SZAngleMax=global, SZAngleMin=global, SZHWidthMax=global, SZHWidthMin=global, SZRange=global, SZRangedot=global, State=global, Warning_Left=global, Warning_Right=global
  wires:
  Bus Selector/1 -> GPS to Relative Position/3(Target lat)  "<Lateral>"
  Bus Selector/2 -> GPS to Relative Position/4(Target long)  "<Longitudinal>"
  GPS to Relative Position/1(Target Range) -> DNPW/1(Range)
  GPS to Relative Position/2(Target Theta) -> DNPW/2(Theta)
  DNPW/1(Left Reminding) -> Mux/1, [Reminding_Left]
  DNPW/3(Left Warning) -> Mux/2, [Warning_Left]
  DNPW/2(Right Reminding) -> Mux1/1, [Reminding_Right]
  DNPW/4(Right Warning) -> Mux1/2, [Warning_Right]
  Mux/1 -> Scope/1  "Left (yellow = reminder; purple = warning)"
  Mux1/1 -> Scope/2  "Right (yellow = reminder; purple = warning)"
  Forward Zone Range [m]/1 -> [FZRange]
  Forward Zone Lane Half Width [m]/1 -> [FZHWidth]
  Forward Zone Angle [deg]/1 -> [FZAngle]
  Side Zone Range [m]/1 -> [SZRange]
  Side Zone Lane Half Width Min [m]/1 -> [SZHWidthMin]
  Side Zone Lane Half Width Max [m]/1 -> [SZHWidthMax]
  SIde Zone Angle Min [deg]/1 -> [SZAngleMin]
  SIde Zone Angle Max [deg]/1 -> [SZAngleMax]
  Side Zone Rangedot [m/s]/1 -> [SZRangedot]
  System Enable Yawrate Threshold [deg/s] </1 -> [SEYawrate]
  System Warning Yawrate Threshold [deg/s] >/1 -> [SWYawrate]
  Gain/1 -> Memory1/1
  SELF_BMW_X5_1/1 -> SELF_Demux/1(SELF)
  DSRC Receiver/1(f()) -> J2735 Decoder Basic Safety Message/Enable
  DSRC Receiver/2(Data) -> J2735 Decoder Basic Safety Message/1(Data)
  DSRC_Rx_1/1 -> DSRC Receiver/1(In1)
  VISUSteer_Mux/1(Steer) -> VISUSteer_BMW_X5_1/1
  Trajectories/1(State) -> STATE_BMW_X5_1/1, [State]
  J2735 Decoder Basic Safety Message/2(Msg) -> Bus Selector/1
  SELF_Demux/12(yaw rate [deg/s]) -> DNPW/3(Yaw Rate), Gain/1
  Constant/1 -> VISUSteer_Mux/1(Column [deg])
  SELF_Demux/11(heading [deg]) -> GPS to Relative Position/5(Host heading)
  SELF_Demux/7(GPS lat [deg]) -> GPS to Relative Position/1(Host lat)
  SELF_Demux/8(GPS long [deg]) -> GPS to Relative Position/2(Host long)
  Memory1/1 -> VISUSteer_Mux/2(Steer [deg])
  J2735 Decoder Basic Safety Message/1(f()) -> Terminator_1/1
  SELF_Demux/1(x [m]) -> Terminator_2/1
  SELF_Demux/2(y [m]) -> Terminator_3/1
  SELF_Demux/3(z [m]) -> Terminator_4/1
  SELF_Demux/4(rotx [deg]) -> Terminator_5/1
  SELF_Demux/5(roty [deg]) -> Terminator_6/1
  SELF_Demux/6(rotz [deg]) -> Terminator_7/1
  SELF_Demux/9(GPS alt [m]) -> Terminator_8/1
  SELF_Demux/10(velocity [m/s]) -> Terminator_9/1

== system Demo_DSRC_DNPW_cs/CollisionDetection ==
  Selector : Selector  IndexMode=Zero-based  IndexOptions=Starting index (dialog)  Indices=PortIndex  OutputSizes=PortWidth(1)
  retrieve CollisionDetection signal : Subsystem
  U : Outport
  U1 : Outport  Port=2
  wires:
  retrieve CollisionDetection signal/1(Out) -> U1/1
  [SimCoreSensors] -> Selector/1
  Selector/1 -> retrieve CollisionDetection signal/1(In), U/1

== system Demo_DSRC_DNPW_cs/DSRC_Rx_1 ==
  Selector : Selector  IndexMode=Zero-based  IndexOptions=Starting index (dialog)  Indices=PortIndex  OutputSizes=PortWidth(1)
  U : Outport
  wires:
  [SimCoreSensors] -> Selector/1
  Selector/1 -> U/1

== system Demo_DSRC_DNPW_cs/DSRC_Tx_1 ==
  Y : Inport  SampleTime=TimeStep
  Assignment : Assignment  IndexMode=Zero-based  SampleTime=TimeStep  IndexOptions=Starting index (dialog)  Indices=PortIndex  OutputSizes=[1 1]
  Data Store Read : DataStoreRead  DataStoreName=SimCoreActuators  SampleTime=TimeStep
  Data Store Write : DataStoreWrite  DataStoreName=SimCoreActuators
  wires:
  Y/1 -> Assignment/2
  Data Store Read/1 -> Assignment/1
  Assignment/1 -> Data Store Write/1

== system Demo_DSRC_DNPW_cs/DSRC_Tx_2 ==
  Y : Inport  SampleTime=TimeStep
  Assignment : Assignment  IndexMode=Zero-based  SampleTime=TimeStep  IndexOptions=Starting index (dialog)  Indices=PortIndex  OutputSizes=[1 1]
  Data Store Read : DataStoreRead  DataStoreName=SimCoreActuators  SampleTime=TimeStep
  Data Store Write : DataStoreWrite  DataStoreName=SimCoreActuators
  wires:
  Y/1 -> Assignment/2
  Data Store Read/1 -> Assignment/1
  Assignment/1 -> Data Store Write/1

== system Demo_DSRC_DNPW_cs/DSRC_Tx_3 ==
  Y : Inport  SampleTime=TimeStep
  Assignment : Assignment  IndexMode=Zero-based  SampleTime=TimeStep  IndexOptions=Starting index (dialog)  Indices=PortIndex  OutputSizes=[1 1]
  Data Store Read : DataStoreRead  DataStoreName=SimCoreActuators  SampleTime=TimeStep
  Data Store Write : DataStoreWrite  DataStoreName=SimCoreActuators
  wires:
  Y/1 -> Assignment/2
  Data Store Read/1 -> Assignment/1
  Assignment/1 -> Data Store Write/1

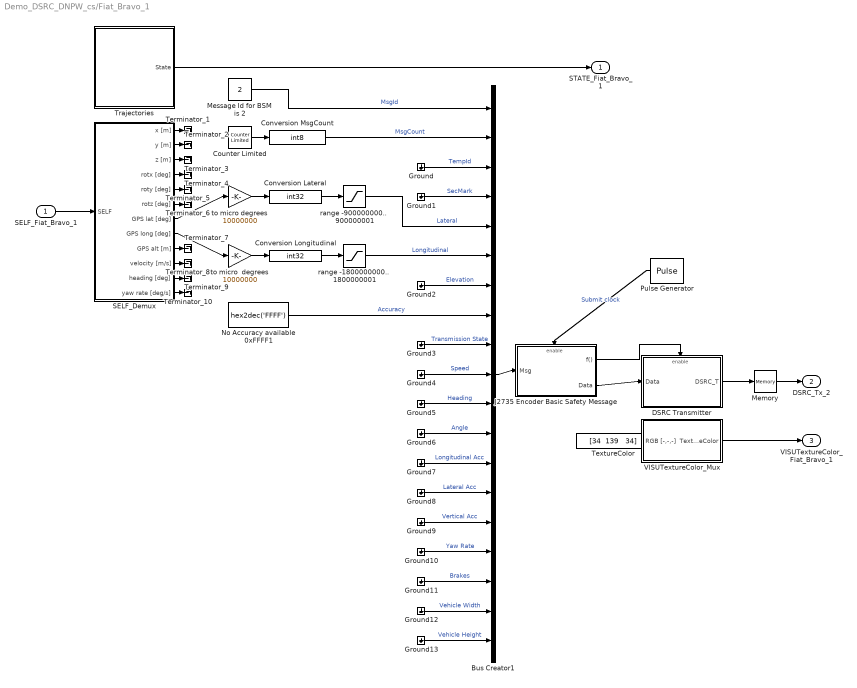
== system Demo_DSRC_DNPW_cs/Fiat_Bravo_1 ==
  SELF_Fiat_Bravo_1 : Inport  Tag=SELFInport
  Bus Creator1 : BusCreator  Inputs=19
  Conversion Lateral : DataTypeConversion  OutDataTypeStr=int32
  Conversion Longitudinal : DataTypeConversion  OutDataTypeStr=int32
  Conversion MsgCount : DataTypeConversion  OutDataTypeStr=int8
  Counter Limited : simulink/Sources/Counter Limited  SystemSampleTime=-1  uplimit=127  tsamp=-1
  DSRC Transmitter : Subsystem  Tag=DSRC_Transmitter
  Ground{,1..13} (14 alike) : Ground
  J2735 Encoder Basic Safety Message : Subsystem  Tag=J2735_Encoder_Basic_Safety_Message
  Memory : Memory
  Message Id for BSM is 2 : Constant  Value=2  OutDataTypeStr=int8
  No Accuracy available 0xFFFF1 : Constant  Value=hex2dec('FFFF')  OutDataTypeStr=int32
  Pulse Generator : DiscretePulseGenerator  Period=1  SampleTime=1/20
  SELF_Demux : Subsystem  Tag=DemuxSELF
      settings: DeleteFcn=PreScanBlockDeleteFcn;
      mask Type: PreScan Demux Block:
      mask Display:
      | port_label('output',1,'x [m]')
      | port_label('output',2,'y [m]')
      | port_label('output',3,'z [m]','texmode','on')
      | port_label('output',4,'Rotx [deg]','texmode','on')
      | port_label('output',5,'Roty [deg]','texmode','on')
      | port_label('output',6,'Rotz [deg]','texmode','on')
      | port_label('output',7,'GPS lat [deg]','texmode','on')
      | port_label('output',8,'GPS long [deg]','texmode','on')
      | port_label('output',9,'GPS alt [m]','texmode','on')
      | port_label('output',10,'Velocity [m/s]')
      | port_label('output',11,'Heading [deg]')
      | port_label('output',12,'Yaw rate [deg/s]')
  Terminator_{1..10} (10 alike) : Terminator
  TextureColor : Constant  Tag=TextureColor  Value="[34  139   34]"
  Trajectories : Subsystem  Tag=Trajectories
      settings: DeleteFcn=PreScanBlockDeleteFcn;
      mask Type: PreScan Source Block: Trajectories
      mask Description:
      | The Trajectory block contains the trajectories defined in the PreScan Experiment Editor. The output of the trajectory block is the (vehicle) State.
      | 
      | For more information, please click Help.
      mask Help: eval('openHelp(312)')
      mask Display: image(imread('Trajectory.png'));
  VISUTextureColor_Mux : Subsystem  Tag=MuxSteer
      settings: DeleteFcn=PreScanBlockDeleteFcn;
      mask Type: PreScan Mux Block:
  range -1800000000..  1800000001 : Saturate  UpperLimit=1800000001  LowerLimit=-1800000000  OutDataTypeStr=int32
  range -900000000..  900000001 : Saturate  UpperLimit=900000001  LowerLimit=-900000000  OutDataTypeStr=int32
  to micro degrees : Gain  Gain=10000000
  to micro  degrees : Gain  Gain=10000000
  STATE_Fiat_Bravo_1 : Outport  Tag=StateOutport
  DSRC_Tx_2 : Outport  Tag=DSRC_TOutport  Port=2
  VISUTextureColor_Fiat_Bravo_1 : Outport  Tag=VisuTextureColorOutport  Port=3  SampleTime=1/20
  wires:
  Message Id for BSM is 2/1 -> Bus Creator1/1  "MsgId"
  Counter Limited/1 -> Conversion MsgCount/1
  to micro  degrees/1 -> Conversion Longitudinal/1
  Conversion Longitudinal/1 -> range -1800000000..  1800000001/1
  Conversion Lateral/1 -> range -900000000..  900000001/1
  to micro degrees/1 -> Conversion Lateral/1
  No Accuracy available 0xFFFF1/1 -> Bus Creator1/8  "Accuracy"
  Ground13/1 -> Bus Creator1/19  "Vehicle Height"
  Ground12/1 -> Bus Creator1/18  "Vehicle Width"
  Ground11/1 -> Bus Creator1/17  "Brakes"
  Ground10/1 -> Bus Creator1/16  "Yaw Rate"
  Ground9/1 -> Bus Creator1/15  "Vertical Acc"
  Ground8/1 -> Bus Creator1/14  "Lateral Acc"
  Ground7/1 -> Bus Creator1/13  "Longitudinal Acc"
  Ground6/1 -> Bus Creator1/12  "Angle"
  Ground2/1 -> Bus Creator1/7  "Elevation"
  Ground1/1 -> Bus Creator1/4  "SecMark"
  Ground/1 -> Bus Creator1/3  "TempId"
  Conversion MsgCount/1 -> Bus Creator1/2  "MsgCount"
  range -900000000..  900000001/1 -> Bus Creator1/5  "Lateral"
  range -1800000000..  1800000001/1 -> Bus Creator1/6  "Longitudinal"
  Ground5/1 -> Bus Creator1/11  "Heading"
  Ground4/1 -> Bus Creator1/10  "Speed"
  Ground3/1 -> Bus Creator1/9  "Transmission State"
  SELF_Fiat_Bravo_1/1 -> SELF_Demux/1(SELF)
  J2735 Encoder Basic Safety Message/1(f()) -> DSRC Transmitter/Enable
  J2735 Encoder Basic Safety Message/2(Data) -> DSRC Transmitter/1(Data)
  DSRC Transmitter/1(DSRC_T) -> Memory/1
  VISUTextureColor_Mux/1(TextureColor) -> VISUTextureColor_Fiat_Bravo_1/1
  TextureColor/1 -> VISUTextureColor_Mux/1(RGB [-,-,-])
  Trajectories/1(State) -> STATE_Fiat_Bravo_1/1
  Bus Creator1/1 -> J2735 Encoder Basic Safety Message/1(Msg)
  Pulse Generator/1 -> J2735 Encoder Basic Safety Message/Enable  "Submit clock"
  SELF_Demux/7(GPS lat [deg]) -> to micro degrees/1
  SELF_Demux/8(GPS long [deg]) -> to micro  degrees/1
  Memory/1 -> DSRC_Tx_2/1
  SELF_Demux/1(x [m]) -> Terminator_1/1
  SELF_Demux/2(y [m]) -> Terminator_2/1
  SELF_Demux/3(z [m]) -> Terminator_3/1
  SELF_Demux/4(rotx [deg]) -> Terminator_4/1
  SELF_Demux/5(roty [deg]) -> Terminator_5/1
  SELF_Demux/6(rotz [deg]) -> Terminator_6/1
  SELF_Demux/9(GPS alt [m]) -> Terminator_7/1
  SELF_Demux/10(velocity [m/s]) -> Terminator_8/1
  SELF_Demux/11(heading [deg]) -> Terminator_9/1
  SELF_Demux/12(yaw rate [deg/s]) -> Terminator_10/1

== system Demo_DSRC_DNPW_cs/GetSensors ==
  dummy : Inport
  GetSensors : M-S-Function  FunctionName=GetSensorsBlock  Parameters=TimeStep NrOfSensors
  tag scope: SimCoreSensors=global
  wires:
  GetSensors/1 -> [SimCoreSensors]
  dummy/1 -> GetSensors/1

== system Demo_DSRC_DNPW_cs/HMI_Box_Left ==
  SELF_HMI_Box_Left : Inport  Tag=SELFInport
  Dynamics_Empty : Subsystem  Tag=Dynamics_Empty
      mask Display: port_label('output', 1, 'State');text(0,0,' Empty\n')
  SELF_Demux : Subsystem  Tag=DemuxSELF
      settings: DeleteFcn=PreScanBlockDeleteFcn;
      mask Type: PreScan Demux Block:
      mask Display:
      | port_label('output',1,'x [m]')
      | port_label('output',2,'y [m]')
      | port_label('output',3,'z [m]','texmode','on')
      | port_label('output',4,'Rotx [deg]','texmode','on')
      | port_label('output',5,'Roty [deg]','texmode','on')
      | port_label('output',6,'Rotz [deg]','texmode','on')
      | port_label('output',7,'GPS lat [deg]','texmode','on')
      | port_label('output',8,'GPS long [deg]','texmode','on')
      | port_label('output',9,'GPS alt [m]','texmode','on')
      | port_label('output',10,'Velocity [m/s]')
      | port_label('output',11,'Heading [deg]')
      | port_label('output',12,'Yaw rate [deg/s]')
  Terminator_{1..13} (13 alike) : Terminator
  STATE_HMI_Box_Left : Outport  Tag=StateOutport
  wires:
  SELF_HMI_Box_Left/1 -> SELF_Demux/1(SELF)
  [State] -> STATE_HMI_Box_Left/1
  Dynamics_Empty/1(State) -> Terminator_1/1
  SELF_Demux/1(x [m]) -> Terminator_2/1
  SELF_Demux/2(y [m]) -> Terminator_3/1
  SELF_Demux/3(z [m]) -> Terminator_4/1
  SELF_Demux/4(rotx [deg]) -> Terminator_5/1
  SELF_Demux/5(roty [deg]) -> Terminator_6/1
  SELF_Demux/6(rotz [deg]) -> Terminator_7/1
  SELF_Demux/7(GPS lat [deg]) -> Terminator_8/1
  SELF_Demux/8(GPS long [deg]) -> Terminator_9/1
  SELF_Demux/9(GPS alt [m]) -> Terminator_10/1
  SELF_Demux/10(velocity [m/s]) -> Terminator_11/1
  SELF_Demux/11(heading [deg]) -> Terminator_12/1
  SELF_Demux/12(yaw rate [deg/s]) -> Terminator_13/1
